simulink model "discon"  (R2018b)
settings: Solver=ode1  StartTime=0.0  StopTime=100  FixedStep=0.1  MaxStep=0.1  RelTol=1e-3
values from neighbouring files (symbols this model uses):
  c1 = 0.000277    [Systemen_mit_Diskontinuty.m]    (also in discontinous.m)
  c2 = 0.00277    [Systemen_mit_Diskontinuty.m]    (also in discontinous.m)
  Fschub1 = 36350.0    (= 36350)    [Systemen_mit_Diskontinuty.m]    (also in discontinous.m)
  Fschub2 = 1308.0    (= 1308)    [Systemen_mit_Diskontinuty.m]    (also in discontinous.m)
  G = 6.67e-11    [Systemen_mit_Diskontinuty.m]    (also in discontinous.m)
  h_thrust_change = 10500.0    (= 10500)    [Systemen_mit_Diskontinuty.m]    (also in discontinous.m)
  M = 7.35e22    (= 7.35e+22)    [Systemen_mit_Diskontinuty.m]    (also in discontinous.m)
  rm = 1738e3    (= 1738000)    [Systemen_mit_Diskontinuty.m]    (also in discontinous.m)
  x1 = 59404.0    (= 59404)    [Systemen_mit_Diskontinuty.m]    (also in discontinous.m)
  x2 = -2003.0    (= -2003)    [Systemen_mit_Diskontinuty.m]    (also in discontinous.m)
  x3 = 1038.358    [Systemen_mit_Diskontinuty.m]    (also in discontinous.m)
libraries: simulink x1
settings Model: Creator=Naveen  LastModifiedBy=Naveen

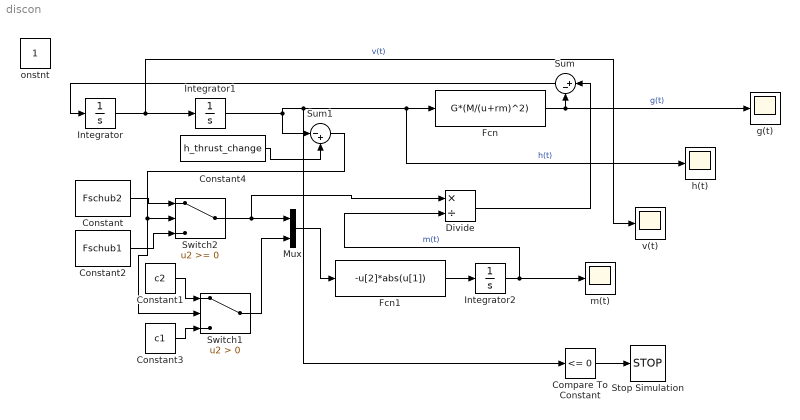
== system discon ==
  Compare To Constant : simulink/Logic and Bit Operations/Compare To Constant  relop=<=  const=0  OutDataTypeStr=boolean
  Constant : Constant  Value=Fschub2
  Constant1 : Constant  Value=c2
  Constant2 : Constant  Value=Fschub1
  Constant3 : Constant  Value=c1
  Constant4 : Constant  Value=h_thrust_change
  Divide : Product  Inputs=*/
  Fcn : Fcn  Expr=G*(M/(u+rm)^2)
  Fcn1 : Fcn  Expr=-u[2]*abs(u[1])
  Integrator : Integrator  InitialCondition=x2
  Integrator1 : Integrator  InitialCondition=x1  LowerSaturationLimit=0
  Integrator2 : Integrator  InitialCondition=x3  LowerSaturationLimit=0
  Mux : Mux  Inputs=2
  Stop Simulation : Stop
  Sum : Sum  Inputs=|+-
  Sum1 : Sum  Inputs=|-+
  Switch1 : Switch  Criteria=u2 > Threshold
  Switch2 : Switch
  g(t) : Scope
  h(t) : Scope
  m(t) : Scope
  v(t) : Scope
  onstnt : Constant  IOType=siggen
  wires:
  Integrator/1 -> v(t)/1, Integrator1/1  "v(t)"
  Constant/1 -> Switch2/1
  Constant2/1 -> Switch2/3
  Constant3/1 -> Switch1/3
  Constant1/1 -> Switch1/1
  Integrator1/1 -> Sum1/1, h(t)/1, Fcn/1, Compare To Constant/1  "h(t)"
  Switch2/1 -> Divide/1, Mux/1
  Switch1/1 -> Mux/2
  Fcn/1 -> g(t)/1, Sum/2  "g(t)"
  Constant4/1 -> Sum1/2
  Sum1/1 -> Switch1/2, Switch2/2
  Mux/1 -> Fcn1/1
  Fcn1/1 -> Integrator2/1
  Integrator2/1 -> m(t)/1, Divide/2  "m(t)"
  Divide/1 -> Sum/1
  Sum/1 -> Integrator/1
  Compare To Constant/1 -> Stop Simulation/1
